simulink model "eyemove1"  (R2014a)
settings: Solver=ode45  StartTime=0.0  StopTime=10.0  RelTol=1e-3
values from neighbouring files (symbols this model uses):
  C1 = 15    [run_eyemove1.m]
  C2 = 25    [run_eyemove1.m]
  K1 = 100    [run_eyemove1.m]
  K2 = 100    [run_eyemove1.m]
  mass = 1    [run_eyemove1.m]
settings Model: ExtModeAutoUpdateStatusClock=off  Creator=mike  LastModifiedBy=jianwang
settings DataIOCC: SignalLoggingSaveFormat=ModelDataLogs  SignalLoggingName=sigsOut
settings DebuggingCC: SaveWithParameterizedLinksMsg=none  UnderspecifiedInitializationDetection=Classic  SignalResolutionControl=TryResolveAllWithWarning  SolverPrmCheckMsg=none  MultiTaskDSMMsg=warning  MultiTaskCondExecSysMsg=none
settings HardwareCC: TargetUnknown=on
settings RTWCC: IncludeERTFirstTime=on
settings GRTTargetCC: CombineOutputUpdateFcns=off  GRTInterface=on

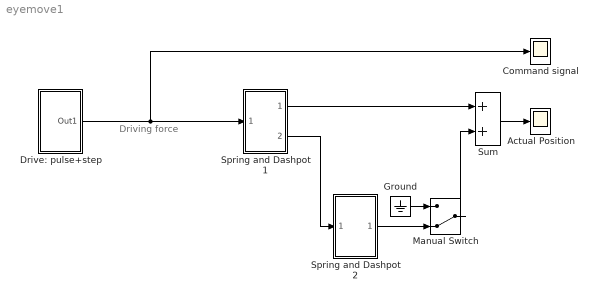
== system eyemove1 ==
  note: Driving force
  Actual Position : Scope
      settings: TickLabels=on  TimeRange=40.000000
  Command signal : Scope
      settings: TickLabels=on  TimeRange=10  YMin=0  YMax=1200
  Drive: pulse+step : Subsystem
  Ground : Ground
  Manual Switch : ManualSwitch  CurrentSetting=0
  Spring and Dashpot 1 : Subsystem
  Spring and Dashpot 2 : Subsystem
  Sum : Sum  SaturateOnIntegerOverflow=on
  wires:
  Drive: pulse+step/1(Out1) -> Command signal/1, Spring and Dashpot 1/1(In1)
  Spring and Dashpot 1/1(Pos) -> Sum/1
  Sum/1 -> Actual Position/1
  Manual Switch/1 -> Sum/2
  Spring and Dashpot 1/2(Force) -> Spring and Dashpot 2/1(In1)
  Ground/1 -> Manual Switch/1
  Spring and Dashpot 2/1(Out1) -> Manual Switch/2

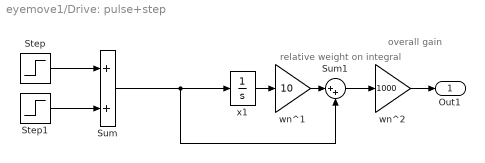
== system eyemove1/Drive: pulse+step ==
  note: relative weight on
      | integral
  note: overall gain
  Step : Step  SampleTime=0
  Step1 : Step  Time=1.05  After=-1  SampleTime=0
  Sum : Sum  SaturateOnIntegerOverflow=on
  Sum1 : Sum  Inputs=|++  SaturateOnIntegerOverflow=on
  wn^1 : Gain  Gain=10  SaturateOnIntegerOverflow=on  OutDataTypeStr=Inherit: Same as input  ParamDataTypeStr=Inherit: Same as input
  wn^2 : Gain  Gain=1000  SaturateOnIntegerOverflow=on  OutDataTypeStr=Inherit: Same as input  ParamDataTypeStr=Inherit: Same as input
  x1 : Integrator
  Out1 : Outport
  wires:
  Sum/1 -> x1/1, Sum1/2
  x1/1 -> wn^1/1
  wn^1/1 -> Sum1/1
  Sum1/1 -> wn^2/1
  wn^2/1 -> Out1/1
  Step/1 -> Sum/1
  Step1/1 -> Sum/2

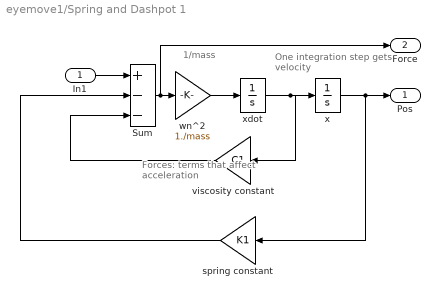
== system eyemove1/Spring and Dashpot 1 ==
  note: 1/mass
  note: Forces: terms that
      | affect acceleration
  note: One integration step
      | gets velocity
  In1 : Inport
  Sum : Sum  Inputs=+--  SaturateOnIntegerOverflow=on  InputSameDT=on  OutDataTypeStr=Inherit: Same as first input
  spring constant : Gain  Gain=K1  SaturateOnIntegerOverflow=on  OutDataTypeStr=Inherit: Same as input  ParamDataTypeStr=Inherit: Same as input
  viscosity constant : Gain  Gain=C1  SaturateOnIntegerOverflow=on  OutDataTypeStr=Inherit: Same as input  ParamDataTypeStr=Inherit: Same as input
  wn^2 : Gain  Gain=1./mass  SaturateOnIntegerOverflow=on  OutDataTypeStr=Inherit: Same as input  ParamDataTypeStr=Inherit: Same as input
  x : Integrator
  xdot : Integrator
  Pos : Outport
  Force : Outport  Port=2
  wires:
  wn^2/1 -> xdot/1
  Sum/1 -> wn^2/1, Force/1
  xdot/1 -> x/1, viscosity constant/1
  x/1 -> spring constant/1, Pos/1
  spring constant/1 -> Sum/2
  viscosity constant/1 -> Sum/3
  In1/1 -> Sum/1

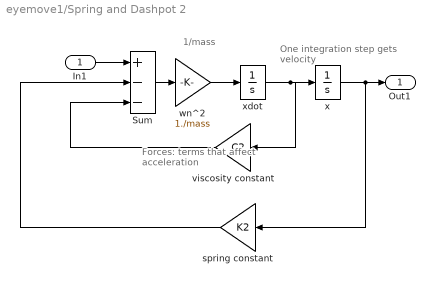
== system eyemove1/Spring and Dashpot 2 ==
  note: 1/mass
  note: Forces: terms that
      | affect acceleration
  note: One integration step
      | gets velocity
  In1 : Inport
  Sum : Sum  Inputs=+--  SaturateOnIntegerOverflow=on  InputSameDT=on  OutDataTypeStr=Inherit: Same as first input
  spring constant : Gain  Gain=K2  SaturateOnIntegerOverflow=on  OutDataTypeStr=Inherit: Same as input  ParamDataTypeStr=Inherit: Same as input
  viscosity constant : Gain  Gain=C2  SaturateOnIntegerOverflow=on  OutDataTypeStr=Inherit: Same as input  ParamDataTypeStr=Inherit: Same as input
  wn^2 : Gain  Gain=1./mass  SaturateOnIntegerOverflow=on  OutDataTypeStr=Inherit: Same as input  ParamDataTypeStr=Inherit: Same as input
  x : Integrator
  xdot : Integrator
  Out1 : Outport
  wires:
  wn^2/1 -> xdot/1
  Sum/1 -> wn^2/1
  xdot/1 -> x/1, viscosity constant/1
  x/1 -> spring constant/1, Out1/1
  spring constant/1 -> Sum/2
  viscosity constant/1 -> Sum/3
  In1/1 -> Sum/1
